simulink model "EHB_speedgoat_R2020a_V1"  (R2020a)
settings: Solver=FixedStepDiscrete  StartTime=0.0  StopTime=inf  FixedStep=0.001  RelTol=1e-3  EnableMultiTasking=on
model workspace (MAT data in the model file):
  A : Simulink.Signal (value not decoded)
  B : Simulink.Signal (value not decoded)
  C : Simulink.Signal (value not decoded)
  D : Simulink.Signal (value not decoded)
  E : Simulink.Signal (value not decoded)
  calin = [-9.96 -7.98 -5.98 -3.99 -1.994 0 1.995 3.992 5.99 7.98 9.97]
  calout = [-10 -8 -6 -4 -2 0 2 4 6 8 10]
symbols that are objects in the model workspace (value not decoded): C, D
undefined symbols (not defined in the file): Com1, none, ts_IO612
libraries: simulink x1436, xpcethercatlib x1223, yisutbxlib_utilities x256, xpcutilitieslib x156, hdlsllib x145, canmsglib x46, speedgoatlib_IO602_4 x11, speedgoatlib_IO611 x7, slrttcplib x4, CanManageLib x3, slrtlib x3, xpcseriallib x2
(part 19 of 30)

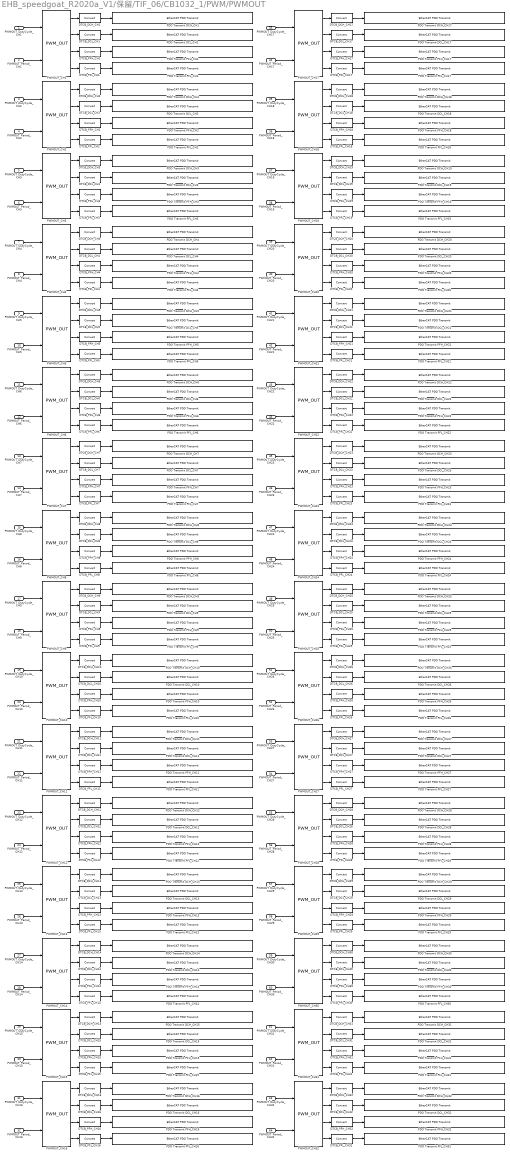
== system EHB_speedgoat_R2020a_V1/保留/TIF_06/CB1032_1/PWM/PWMOUT ==
  PWMOUT_DutyCycle_CH1 : Inport
  PWMOUT_Period_CH1 : Inport  Port=2
  PWMOUT_DutyCycle_CH2 : Inport  Port=3
  PWMOUT_Period_CH2 : Inport  Port=4
  PWMOUT_DutyCycle_CH3 : Inport  Port=5
  PWMOUT_Period_CH3 : Inport  Port=6
  PWMOUT_DutyCycle_CH4 : Inport  Port=7
  PWMOUT_Period_CH4 : Inport  Port=8
  PWMOUT_DutyCycle_CH5 : Inport  Port=9
  PWMOUT_Period_CH5 : Inport  Port=10
  PWMOUT_DutyCycle_CH6 : Inport  Port=11
  PWMOUT_Period_CH6 : Inport  Port=12
  PWMOUT_DutyCycle_CH7 : Inport  Port=13
  PWMOUT_Period_CH7 : Inport  Port=14
  PWMOUT_DutyCycle_CH8 : Inport  Port=15
  PWMOUT_Period_CH8 : Inport  Port=16
  PWMOUT_DutyCycle_CH9 : Inport  Port=17
  PWMOUT_Period_CH9 : Inport  Port=18
  PWMOUT_DutyCycle_CH10 : Inport  Port=19
  PWMOUT_Period_CH10 : Inport  Port=20
  PWMOUT_DutyCycle_CH11 : Inport  Port=21
  PWMOUT_Period_CH11 : Inport  Port=22
  PWMOUT_DutyCycle_CH12 : Inport  Port=23
  PWMOUT_Period_CH12 : Inport  Port=24
  PWMOUT_DutyCycle_CH13 : Inport  Port=25
  PWMOUT_Period_CH13 : Inport  Port=26
  PWMOUT_DutyCycle_CH14 : Inport  Port=27
  PWMOUT_Period_CH14 : Inport  Port=28
  PWMOUT_DutyCycle_CH15 : Inport  Port=29
  PWMOUT_Period_CH15 : Inport  Port=30
  PWMOUT_DutyCycle_CH16 : Inport  Port=31
  PWMOUT_Period_CH16 : Inport  Port=32
  PWMOUT_DutyCycle_CH17 : Inport  Port=33
  PWMOUT_Period_CH17 : Inport  Port=34
  PWMOUT_DutyCycle_CH18 : Inport  Port=35
  PWMOUT_Period_CH18 : Inport  Port=36
  PWMOUT_DutyCycle_CH19 : Inport  Port=37
  PWMOUT_Period_CH19 : Inport  Port=38
  PWMOUT_DutyCycle_CH20 : Inport  Port=39
  PWMOUT_Period_CH20 : Inport  Port=40
  PWMOUT_DutyCycle_CH21 : Inport  Port=41
  PWMOUT_Period_CH21 : Inport  Port=42
  PWMOUT_DutyCycle_CH22 : Inport  Port=43
  PWMOUT_Period_CH22 : Inport  Port=44
  PWMOUT_DutyCycle_CH23 : Inport  Port=45
  PWMOUT_Period_CH23 : Inport  Port=46
  PWMOUT_DutyCycle_CH24 : Inport  Port=47
  PWMOUT_Period_CH24 : Inport  Port=48
  PWMOUT_DutyCycle_CH25 : Inport  Port=49
  PWMOUT_Period_CH25 : Inport  Port=50
  PWMOUT_DutyCycle_CH26 : Inport  Port=51
  PWMOUT_Period_CH26 : Inport  Port=52
  PWMOUT_DutyCycle_CH27 : Inport  Port=53
  PWMOUT_Period_CH27 : Inport  Port=54
  PWMOUT_DutyCycle_CH28 : Inport  Port=55
  PWMOUT_Period_CH28 : Inport  Port=56
  PWMOUT_DutyCycle_CH29 : Inport  Port=57
  PWMOUT_Period_CH29 : Inport  Port=58
  PWMOUT_DutyCycle_CH30 : Inport  Port=59
  PWMOUT_Period_CH30 : Inport  Port=60
  PWMOUT_DutyCycle_CH31 : Inport  Port=61
  PWMOUT_Period_CH31 : Inport  Port=62
  PWMOUT_DutyCycle_CH32 : Inport  Port=63
  PWMOUT_Period_CH32 : Inport  Port=64
  DTCB_DCH_CH{1..32} (32 alike) : DataTypeConversion
  DTCB_DCL_CH{1..32} (32 alike) : DataTypeConversion
  DTCB_PFH_CH{1..32} (32 alike) : DataTypeConversion
  DTCB_PFL_CH{1..32} (32 alike) : DataTypeConversion
  PDO Transmit DCH_CH1 : xpcethercatlib/EtherCAT PDO Transmit   Priority=3  sig_name=Box 1 (YISUWORLD_Dig).PDOSet1 process data mapping.DCH1  sig_offset=376  sig_type=uint16  type_size=16  sig_dim=1  device_id=0  sample_time=0.001000
      settings: SourceProductBaseCode=XP
  PDO Transmit DCH_CH10 : xpcethercatlib/EtherCAT PDO Transmit   Priority=3  sig_name=Box 1 (YISUWORLD_Dig).PDOSet1 process data mapping.DCH10  sig_offset=520  sig_type=uint16  type_size=16  sig_dim=1  device_id=0  sample_time=0.001000
      settings: SourceProductBaseCode=XP
  PDO Transmit DCH_CH11 : xpcethercatlib/EtherCAT PDO Transmit   Priority=3  sig_name=Box 1 (YISUWORLD_Dig).PDOSet1 process data mapping.DCH11  sig_offset=536  sig_type=uint16  type_size=16  sig_dim=1  device_id=0  sample_time=0.001000
      settings: SourceProductBaseCode=XP
  PDO Transmit DCH_CH12 : xpcethercatlib/EtherCAT PDO Transmit   Priority=3  sig_name=Box 1 (YISUWORLD_Dig).PDOSet1 process data mapping.DCH12  sig_offset=552  sig_type=uint16  type_size=16  sig_dim=1  device_id=0  sample_time=0.001000
      settings: SourceProductBaseCode=XP
  PDO Transmit DCH_CH13 : xpcethercatlib/EtherCAT PDO Transmit   Priority=3  sig_name=Box 1 (YISUWORLD_Dig).PDOSet1 process data mapping.DCH13  sig_offset=568  sig_type=uint16  type_size=16  sig_dim=1  device_id=0  sample_time=0.001000
      settings: SourceProductBaseCode=XP
  PDO Transmit DCH_CH14 : xpcethercatlib/EtherCAT PDO Transmit   Priority=3  sig_name=Box 1 (YISUWORLD_Dig).PDOSet1 process data mapping.DCH14  sig_offset=584  sig_type=uint16  type_size=16  sig_dim=1  device_id=0  sample_time=0.001000
      settings: SourceProductBaseCode=XP
  PDO Transmit DCH_CH15 : xpcethercatlib/EtherCAT PDO Transmit   Priority=3  sig_name=Box 1 (YISUWORLD_Dig).PDOSet1 process data mapping.DCH15  sig_offset=600  sig_type=uint16  type_size=16  sig_dim=1  device_id=0  sample_time=0.001000
      settings: SourceProductBaseCode=XP
  PDO Transmit DCH_CH16 : xpcethercatlib/EtherCAT PDO Transmit   Priority=3  sig_name=Box 1 (YISUWORLD_Dig).PDOSet1 process data mapping.DCH16  sig_offset=616  sig_type=uint16  type_size=16  sig_dim=1  device_id=0  sample_time=0.001000
      settings: SourceProductBaseCode=XP
  PDO Transmit DCH_CH17 : xpcethercatlib/EtherCAT PDO Transmit   Priority=3  sig_name=Box 1 (YISUWORLD_Dig).PDOSet1 process data mapping.DCH17  sig_offset=632  sig_type=uint16  type_size=16  sig_dim=1  device_id=0  sample_time=0.001000
      settings: SourceProductBaseCode=XP
  PDO Transmit DCH_CH18 : xpcethercatlib/EtherCAT PDO Transmit   Priority=3  sig_name=Box 1 (YISUWORLD_Dig).PDOSet1 process data mapping.DCH18  sig_offset=648  sig_type=uint16  type_size=16  sig_dim=1  device_id=0  sample_time=0.001000
      settings: SourceProductBaseCode=XP
  PDO Transmit DCH_CH19 : xpcethercatlib/EtherCAT PDO Transmit   Priority=3  sig_name=Box 1 (YISUWORLD_Dig).PDOSet1 process data mapping.DCH19  sig_offset=664  sig_type=uint16  type_size=16  sig_dim=1  device_id=0  sample_time=0.001000
      settings: SourceProductBaseCode=XP
  PDO Transmit DCH_CH2 : xpcethercatlib/EtherCAT PDO Transmit   Priority=3  sig_name=Box 1 (YISUWORLD_Dig).PDOSet1 process data mapping.DCH2  sig_offset=392  sig_type=uint16  type_size=16  sig_dim=1  device_id=0  sample_time=0.001000
      settings: SourceProductBaseCode=XP
  PDO Transmit DCH_CH20 : xpcethercatlib/EtherCAT PDO Transmit   Priority=3  sig_name=Box 1 (YISUWORLD_Dig).PDOSet1 process data mapping.DCH20  sig_offset=680  sig_type=uint16  type_size=16  sig_dim=1  device_id=0  sample_time=0.001000
      settings: SourceProductBaseCode=XP
  PDO Transmit DCH_CH21 : xpcethercatlib/EtherCAT PDO Transmit   Priority=3  sig_name=Box 1 (YISUWORLD_Dig).PDOSet1 process data mapping.DCH21  sig_offset=696  sig_type=uint16  type_size=16  sig_dim=1  device_id=0  sample_time=0.001000
      settings: SourceProductBaseCode=XP
  PDO Transmit DCH_CH22 : xpcethercatlib/EtherCAT PDO Transmit   Priority=3  sig_name=Box 1 (YISUWORLD_Dig).PDOSet1 process data mapping.DCH22  sig_offset=712  sig_type=uint16  type_size=16  sig_dim=1  device_id=0  sample_time=0.001000
      settings: SourceProductBaseCode=XP
  PDO Transmit DCH_CH23 : xpcethercatlib/EtherCAT PDO Transmit   Priority=3  sig_name=Box 1 (YISUWORLD_Dig).PDOSet1 process data mapping.DCH23  sig_offset=728  sig_type=uint16  type_size=16  sig_dim=1  device_id=0  sample_time=0.001000
      settings: SourceProductBaseCode=XP
  PDO Transmit DCH_CH24 : xpcethercatlib/EtherCAT PDO Transmit   Priority=3  sig_name=Box 1 (YISUWORLD_Dig).PDOSet1 process data mapping.DCH24  sig_offset=744  sig_type=uint16  type_size=16  sig_dim=1  device_id=0  sample_time=0.001000
      settings: SourceProductBaseCode=XP
  PDO Transmit DCH_CH25 : xpcethercatlib/EtherCAT PDO Transmit   Priority=3  sig_name=Box 1 (YISUWORLD_Dig).PDOSet1 process data mapping.DCH25  sig_offset=760  sig_type=uint16  type_size=16  sig_dim=1  device_id=0  sample_time=0.001000
      settings: SourceProductBaseCode=XP
  PDO Transmit DCH_CH26 : xpcethercatlib/EtherCAT PDO Transmit   Priority=3  sig_name=Box 1 (YISUWORLD_Dig).PDOSet1 process data mapping.DCH26  sig_offset=776  sig_type=uint16  type_size=16  sig_dim=1  device_id=0  sample_time=0.001000
      settings: SourceProductBaseCode=XP
  PDO Transmit DCH_CH27 : xpcethercatlib/EtherCAT PDO Transmit   Priority=3  sig_name=Box 1 (YISUWORLD_Dig).PDOSet1 process data mapping.DCH27  sig_offset=792  sig_type=uint16  type_size=16  sig_dim=1  device_id=0  sample_time=0.001000
      settings: SourceProductBaseCode=XP
  PDO Transmit DCH_CH28 : xpcethercatlib/EtherCAT PDO Transmit   Priority=3  sig_name=Box 1 (YISUWORLD_Dig).PDOSet1 process data mapping.DCH28  sig_offset=808  sig_type=uint16  type_size=16  sig_dim=1  device_id=0  sample_time=0.001000
      settings: SourceProductBaseCode=XP
  PDO Transmit DCH_CH29 : xpcethercatlib/EtherCAT PDO Transmit   Priority=3  sig_name=Box 1 (YISUWORLD_Dig).PDOSet1 process data mapping.DCH29  sig_offset=824  sig_type=uint16  type_size=16  sig_dim=1  device_id=0  sample_time=0.001000
      settings: SourceProductBaseCode=XP
  PDO Transmit DCH_CH3 : xpcethercatlib/EtherCAT PDO Transmit   Priority=3  sig_name=Box 1 (YISUWORLD_Dig).PDOSet1 process data mapping.DCH3  sig_offset=408  sig_type=uint16  type_size=16  sig_dim=1  device_id=0  sample_time=0.001000
      settings: SourceProductBaseCode=XP
  PDO Transmit DCH_CH30 : xpcethercatlib/EtherCAT PDO Transmit   Priority=3  sig_name=Box 1 (YISUWORLD_Dig).PDOSet1 process data mapping.DCH30  sig_offset=840  sig_type=uint16  type_size=16  sig_dim=1  device_id=0  sample_time=0.001000
      settings: SourceProductBaseCode=XP
  PDO Transmit DCH_CH31 : xpcethercatlib/EtherCAT PDO Transmit   Priority=3  sig_name=Box 1 (YISUWORLD_Dig).PDOSet1 process data mapping.DCH31  sig_offset=856  sig_type=uint16  type_size=16  sig_dim=1  device_id=0  sample_time=0.001000
      settings: SourceProductBaseCode=XP
  PDO Transmit DCH_CH32 : xpcethercatlib/EtherCAT PDO Transmit   Priority=3  sig_name=Box 1 (YISUWORLD_Dig).PDOSet1 process data mapping.DCH32  sig_offset=872  sig_type=uint16  type_size=16  sig_dim=1  device_id=0  sample_time=0.001000
      settings: SourceProductBaseCode=XP
  PDO Transmit DCH_CH4 : xpcethercatlib/EtherCAT PDO Transmit   Priority=3  sig_name=Box 1 (YISUWORLD_Dig).PDOSet1 process data mapping.DCH4  sig_offset=424  sig_type=uint16  type_size=16  sig_dim=1  device_id=0  sample_time=0.001000
      settings: SourceProductBaseCode=XP
  PDO Transmit DCH_CH5 : xpcethercatlib/EtherCAT PDO Transmit   Priority=3  sig_name=Box 1 (YISUWORLD_Dig).PDOSet1 process data mapping.DCH5  sig_offset=440  sig_type=uint16  type_size=16  sig_dim=1  device_id=0  sample_time=0.001000
      settings: SourceProductBaseCode=XP
  PDO Transmit DCH_CH6 : xpcethercatlib/EtherCAT PDO Transmit   Priority=3  sig_name=Box 1 (YISUWORLD_Dig).PDOSet1 process data mapping.DCH6  sig_offset=456  sig_type=uint16  type_size=16  sig_dim=1  device_id=0  sample_time=0.001000
      settings: SourceProductBaseCode=XP
  PDO Transmit DCH_CH7 : xpcethercatlib/EtherCAT PDO Transmit   Priority=3  sig_name=Box 1 (YISUWORLD_Dig).PDOSet1 process data mapping.DCH7  sig_offset=472  sig_type=uint16  type_size=16  sig_dim=1  device_id=0  sample_time=0.001000
      settings: SourceProductBaseCode=XP
  PDO Transmit DCH_CH8 : xpcethercatlib/EtherCAT PDO Transmit   Priority=3  sig_name=Box 1 (YISUWORLD_Dig).PDOSet1 process data mapping.DCH8  sig_offset=488  sig_type=uint16  type_size=16  sig_dim=1  device_id=0  sample_time=0.001000
      settings: SourceProductBaseCode=XP
  PDO Transmit DCH_CH9 : xpcethercatlib/EtherCAT PDO Transmit   Priority=3  sig_name=Box 1 (YISUWORLD_Dig).PDOSet1 process data mapping.DCH9  sig_offset=504  sig_type=uint16  type_size=16  sig_dim=1  device_id=0  sample_time=0.001000
      settings: SourceProductBaseCode=XP
  PDO Transmit DCL_CH1 : xpcethercatlib/EtherCAT PDO Transmit   Priority=3  sig_name=Box 1 (YISUWORLD_Dig).PDOSet1 process data mapping.DCL1  sig_offset=888  sig_type=uint16  type_size=16  sig_dim=1  device_id=0  sample_time=0.001000
      settings: SourceProductBaseCode=XP
  PDO Transmit DCL_CH10 : xpcethercatlib/EtherCAT PDO Transmit   Priority=3  sig_name=Box 1 (YISUWORLD_Dig).PDOSet1 process data mapping.DCL10  sig_offset=1032  sig_type=uint16  type_size=16  sig_dim=1  device_id=0  sample_time=0.001000
      settings: SourceProductBaseCode=XP
  PDO Transmit DCL_CH11 : xpcethercatlib/EtherCAT PDO Transmit   Priority=3  sig_name=Box 1 (YISUWORLD_Dig).PDOSet1 process data mapping.DCL11  sig_offset=1048  sig_type=uint16  type_size=16  sig_dim=1  device_id=0  sample_time=0.001000
      settings: SourceProductBaseCode=XP
  PDO Transmit DCL_CH12 : xpcethercatlib/EtherCAT PDO Transmit   Priority=3  sig_name=Box 1 (YISUWORLD_Dig).PDOSet1 process data mapping.DCL12  sig_offset=1064  sig_type=uint16  type_size=16  sig_dim=1  device_id=0  sample_time=0.001000
      settings: SourceProductBaseCode=XP
  PDO Transmit DCL_CH13 : xpcethercatlib/EtherCAT PDO Transmit   Priority=3  sig_name=Box 1 (YISUWORLD_Dig).PDOSet1 process data mapping.DCL13  sig_offset=1080  sig_type=uint16  type_size=16  sig_dim=1  device_id=0  sample_time=0.001000
      settings: SourceProductBaseCode=XP
  PDO Transmit DCL_CH14 : xpcethercatlib/EtherCAT PDO Transmit   Priority=3  sig_name=Box 1 (YISUWORLD_Dig).PDOSet1 process data mapping.DCL14  sig_offset=1096  sig_type=uint16  type_size=16  sig_dim=1  device_id=0  sample_time=0.001000
      settings: SourceProductBaseCode=XP
  PDO Transmit DCL_CH15 : xpcethercatlib/EtherCAT PDO Transmit   Priority=3  sig_name=Box 1 (YISUWORLD_Dig).PDOSet1 process data mapping.DCL15  sig_offset=1112  sig_type=uint16  type_size=16  sig_dim=1  device_id=0  sample_time=0.001000
      settings: SourceProductBaseCode=XP
  PDO Transmit DCL_CH16 : xpcethercatlib/EtherCAT PDO Transmit   Priority=3  sig_name=Box 1 (YISUWORLD_Dig).PDOSet1 process data mapping.DCL16  sig_offset=1128  sig_type=uint16  type_size=16  sig_dim=1  device_id=0  sample_time=0.001000
      settings: SourceProductBaseCode=XP
  PDO Transmit DCL_CH17 : xpcethercatlib/EtherCAT PDO Transmit   Priority=3  sig_name=Box 1 (YISUWORLD_Dig).PDOSet1 process data mapping.DCL17  sig_offset=1144  sig_type=uint16  type_size=16  sig_dim=1  device_id=0  sample_time=0.001000
      settings: SourceProductBaseCode=XP
  PDO Transmit DCL_CH18 : xpcethercatlib/EtherCAT PDO Transmit   Priority=3  sig_name=Box 1 (YISUWORLD_Dig).PDOSet1 process data mapping.DCL18  sig_offset=1160  sig_type=uint16  type_size=16  sig_dim=1  device_id=0  sample_time=0.001000
      settings: SourceProductBaseCode=XP
  PDO Transmit DCL_CH19 : xpcethercatlib/EtherCAT PDO Transmit   Priority=3  sig_name=Box 1 (YISUWORLD_Dig).PDOSet1 process data mapping.DCL19  sig_offset=1176  sig_type=uint16  type_size=16  sig_dim=1  device_id=0  sample_time=0.001000
      settings: SourceProductBaseCode=XP
  PDO Transmit DCL_CH2 : xpcethercatlib/EtherCAT PDO Transmit   Priority=3  sig_name=Box 1 (YISUWORLD_Dig).PDOSet1 process data mapping.DCL2  sig_offset=904  sig_type=uint16  type_size=16  sig_dim=1  device_id=0  sample_time=0.001000
      settings: SourceProductBaseCode=XP
  PDO Transmit DCL_CH20 : xpcethercatlib/EtherCAT PDO Transmit   Priority=3  sig_name=Box 1 (YISUWORLD_Dig).PDOSet1 process data mapping.DCL20  sig_offset=1192  sig_type=uint16  type_size=16  sig_dim=1  device_id=0  sample_time=0.001000
      settings: SourceProductBaseCode=XP
  PDO Transmit DCL_CH21 : xpcethercatlib/EtherCAT PDO Transmit   Priority=3  sig_name=Box 1 (YISUWORLD_Dig).PDOSet1 process data mapping.DCL21  sig_offset=1208  sig_type=uint16  type_size=16  sig_dim=1  device_id=0  sample_time=0.001000
      settings: SourceProductBaseCode=XP
  PDO Transmit DCL_CH22 : xpcethercatlib/EtherCAT PDO Transmit   Priority=3  sig_name=Box 1 (YISUWORLD_Dig).PDOSet1 process data mapping.DCL22  sig_offset=1224  sig_type=uint16  type_size=16  sig_dim=1  device_id=0  sample_time=0.001000
      settings: SourceProductBaseCode=XP
  PDO Transmit DCL_CH23 : xpcethercatlib/EtherCAT PDO Transmit   Priority=3  sig_name=Box 1 (YISUWORLD_Dig).PDOSet1 process data mapping.DCL23  sig_offset=1240  sig_type=uint16  type_size=16  sig_dim=1  device_id=0  sample_time=0.001000
      settings: SourceProductBaseCode=XP
  PDO Transmit DCL_CH24 : xpcethercatlib/EtherCAT PDO Transmit   Priority=3  sig_name=Box 1 (YISUWORLD_Dig).PDOSet1 process data mapping.DCL24  sig_offset=1256  sig_type=uint16  type_size=16  sig_dim=1  device_id=0  sample_time=0.001000
      settings: SourceProductBaseCode=XP
  PDO Transmit DCL_CH25 : xpcethercatlib/EtherCAT PDO Transmit   Priority=3  sig_name=Box 1 (YISUWORLD_Dig).PDOSet1 process data mapping.DCL25  sig_offset=1272  sig_type=uint16  type_size=16  sig_dim=1  device_id=0  sample_time=0.001000
      settings: SourceProductBaseCode=XP
  PDO Transmit DCL_CH26 : xpcethercatlib/EtherCAT PDO Transmit   Priority=3  sig_name=Box 1 (YISUWORLD_Dig).PDOSet1 process data mapping.DCL26  sig_offset=1288  sig_type=uint16  type_size=16  sig_dim=1  device_id=0  sample_time=0.001000
      settings: SourceProductBaseCode=XP
  PDO Transmit DCL_CH27 : xpcethercatlib/EtherCAT PDO Transmit   Priority=3  sig_name=Box 1 (YISUWORLD_Dig).PDOSet1 process data mapping.DCL27  sig_offset=1304  sig_type=uint16  type_size=16  sig_dim=1  device_id=0  sample_time=0.001000
      settings: SourceProductBaseCode=XP
  PDO Transmit DCL_CH28 : xpcethercatlib/EtherCAT PDO Transmit   Priority=3  sig_name=Box 1 (YISUWORLD_Dig).PDOSet1 process data mapping.DCL28  sig_offset=1320  sig_type=uint16  type_size=16  sig_dim=1  device_id=0  sample_time=0.001000
      settings: SourceProductBaseCode=XP
  PDO Transmit DCL_CH29 : xpcethercatlib/EtherCAT PDO Transmit   Priority=3  sig_name=Box 1 (YISUWORLD_Dig).PDOSet1 process data mapping.DCL29  sig_offset=1336  sig_type=uint16  type_size=16  sig_dim=1  device_id=0  sample_time=0.001000
      settings: SourceProductBaseCode=XP
  PDO Transmit DCL_CH3 : xpcethercatlib/EtherCAT PDO Transmit   Priority=3  sig_name=Box 1 (YISUWORLD_Dig).PDOSet1 process data mapping.DCL3  sig_offset=920  sig_type=uint16  type_size=16  sig_dim=1  device_id=0  sample_time=0.001000
      settings: SourceProductBaseCode=XP
  PDO Transmit DCL_CH30 : xpcethercatlib/EtherCAT PDO Transmit   Priority=3  sig_name=Box 1 (YISUWORLD_Dig).PDOSet1 process data mapping.DCL30  sig_offset=1352  sig_type=uint16  type_size=16  sig_dim=1  device_id=0  sample_time=0.001000
      settings: SourceProductBaseCode=XP
  PDO Transmit DCL_CH31 : xpcethercatlib/EtherCAT PDO Transmit   Priority=3  sig_name=Box 1 (YISUWORLD_Dig).PDOSet1 process data mapping.DCL31  sig_offset=1368  sig_type=uint16  type_size=16  sig_dim=1  device_id=0  sample_time=0.001000
      settings: SourceProductBaseCode=XP
  PDO Transmit DCL_CH32 : xpcethercatlib/EtherCAT PDO Transmit   Priority=3  sig_name=Box 1 (YISUWORLD_Dig).PDOSet1 process data mapping.DCL32  sig_offset=1384  sig_type=uint16  type_size=16  sig_dim=1  device_id=0  sample_time=0.001000
      settings: SourceProductBaseCode=XP
  PDO Transmit DCL_CH4 : xpcethercatlib/EtherCAT PDO Transmit   Priority=3  sig_name=Box 1 (YISUWORLD_Dig).PDOSet1 process data mapping.DCL4  sig_offset=936  sig_type=uint16  type_size=16  sig_dim=1  device_id=0  sample_time=0.001000
      settings: SourceProductBaseCode=XP
  PDO Transmit DCL_CH5 : xpcethercatlib/EtherCAT PDO Transmit   Priority=3  sig_name=Box 1 (YISUWORLD_Dig).PDOSet1 process data mapping.DCL5  sig_offset=952  sig_type=uint16  type_size=16  sig_dim=1  device_id=0  sample_time=0.001000
      settings: SourceProductBaseCode=XP
  PDO Transmit DCL_CH6 : xpcethercatlib/EtherCAT PDO Transmit   Priority=3  sig_name=Box 1 (YISUWORLD_Dig).PDOSet1 process data mapping.DCL6  sig_offset=968  sig_type=uint16  type_size=16  sig_dim=1  device_id=0  sample_time=0.001000
      settings: SourceProductBaseCode=XP
  PDO Transmit DCL_CH7 : xpcethercatlib/EtherCAT PDO Transmit   Priority=3  sig_name=Box 1 (YISUWORLD_Dig).PDOSet1 process data mapping.DCL7  sig_offset=984  sig_type=uint16  type_size=16  sig_dim=1  device_id=0  sample_time=0.001000
      settings: SourceProductBaseCode=XP
  PDO Transmit DCL_CH8 : xpcethercatlib/EtherCAT PDO Transmit   Priority=3  sig_name=Box 1 (YISUWORLD_Dig).PDOSet1 process data mapping.DCL8  sig_offset=1000  sig_type=uint16  type_size=16  sig_dim=1  device_id=0  sample_time=0.001000
      settings: SourceProductBaseCode=XP
  PDO Transmit DCL_CH9 : xpcethercatlib/EtherCAT PDO Transmit   Priority=3  sig_name=Box 1 (YISUWORLD_Dig).PDOSet1 process data mapping.DCL9  sig_offset=1016  sig_type=uint16  type_size=16  sig_dim=1  device_id=0  sample_time=0.001000
      settings: SourceProductBaseCode=XP
  PDO Transmit PFH_CH1 : xpcethercatlib/EtherCAT PDO Transmit   Priority=3  sig_name=Box 1 (YISUWORLD_Dig).PDOSet1 process data mapping.PFH1  sig_offset=1400  sig_type=uint16  type_size=16  sig_dim=1  device_id=0  sample_time=0.001000
      settings: SourceProductBaseCode=XP
  PDO Transmit PFH_CH10 : xpcethercatlib/EtherCAT PDO Transmit   Priority=3  sig_name=Box 1 (YISUWORLD_Dig).PDOSet1 process data mapping.PFH10  sig_offset=1544  sig_type=uint16  type_size=16  sig_dim=1  device_id=0  sample_time=0.001000
      settings: SourceProductBaseCode=XP
  PDO Transmit PFH_CH11 : xpcethercatlib/EtherCAT PDO Transmit   Priority=3  sig_name=Box 1 (YISUWORLD_Dig).PDOSet1 process data mapping.PFH11  sig_offset=1560  sig_type=uint16  type_size=16  sig_dim=1  device_id=0  sample_time=0.001000
      settings: SourceProductBaseCode=XP
  PDO Transmit PFH_CH12 : xpcethercatlib/EtherCAT PDO Transmit   Priority=3  sig_name=Box 1 (YISUWORLD_Dig).PDOSet1 process data mapping.PFH12  sig_offset=1576  sig_type=uint16  type_size=16  sig_dim=1  device_id=0  sample_time=0.001000
      settings: SourceProductBaseCode=XP
  PDO Transmit PFH_CH13 : xpcethercatlib/EtherCAT PDO Transmit   Priority=3  sig_name=Box 1 (YISUWORLD_Dig).PDOSet1 process data mapping.PFH13  sig_offset=1592  sig_type=uint16  type_size=16  sig_dim=1  device_id=0  sample_time=0.001000
      settings: SourceProductBaseCode=XP
  PDO Transmit PFH_CH14 : xpcethercatlib/EtherCAT PDO Transmit   Priority=3  sig_name=Box 1 (YISUWORLD_Dig).PDOSet1 process data mapping.PFH14  sig_offset=1608  sig_type=uint16  type_size=16  sig_dim=1  device_id=0  sample_time=0.001000
      settings: SourceProductBaseCode=XP
  PDO Transmit PFH_CH15 : xpcethercatlib/EtherCAT PDO Transmit   Priority=3  sig_name=Box 1 (YISUWORLD_Dig).PDOSet1 process data mapping.PFH15  sig_offset=1624  sig_type=uint16  type_size=16  sig_dim=1  device_id=0  sample_time=0.001000
      settings: SourceProductBaseCode=XP
  PDO Transmit PFH_CH16 : xpcethercatlib/EtherCAT PDO Transmit   Priority=3  sig_name=Box 1 (YISUWORLD_Dig).PDOSet1 process data mapping.PFH16  sig_offset=1640  sig_type=uint16  type_size=16  sig_dim=1  device_id=0  sample_time=0.001000
      settings: SourceProductBaseCode=XP
  PDO Transmit PFH_CH17 : xpcethercatlib/EtherCAT PDO Transmit   Priority=3  sig_name=Box 1 (YISUWORLD_Dig).PDOSet1 process data mapping.PFH17  sig_offset=1656  sig_type=uint16  type_size=16  sig_dim=1  device_id=0  sample_time=0.001000
      settings: SourceProductBaseCode=XP
  PDO Transmit PFH_CH18 : xpcethercatlib/EtherCAT PDO Transmit   Priority=3  sig_name=Box 1 (YISUWORLD_Dig).PDOSet1 process data mapping.PFH18  sig_offset=1672  sig_type=uint16  type_size=16  sig_dim=1  device_id=0  sample_time=0.001000
      settings: SourceProductBaseCode=XP
  PDO Transmit PFH_CH19 : xpcethercatlib/EtherCAT PDO Transmit   Priority=3  sig_name=Box 1 (YISUWORLD_Dig).PDOSet1 process data mapping.PFH19  sig_offset=1688  sig_type=uint16  type_size=16  sig_dim=1  device_id=0  sample_time=0.001000
      settings: SourceProductBaseCode=XP
  PDO Transmit PFH_CH2 : xpcethercatlib/EtherCAT PDO Transmit   Priority=3  sig_name=Box 1 (YISUWORLD_Dig).PDOSet1 process data mapping.PFH2  sig_offset=1416  sig_type=uint16  type_size=16  sig_dim=1  device_id=0  sample_time=0.001000
      settings: SourceProductBaseCode=XP
  PDO Transmit PFH_CH20 : xpcethercatlib/EtherCAT PDO Transmit   Priority=3  sig_name=Box 1 (YISUWORLD_Dig).PDOSet1 process data mapping.PFH20  sig_offset=1704  sig_type=uint16  type_size=16  sig_dim=1  device_id=0  sample_time=0.001000
      settings: SourceProductBaseCode=XP
  PDO Transmit PFH_CH21 : xpcethercatlib/EtherCAT PDO Transmit   Priority=3  sig_name=Box 1 (YISUWORLD_Dig).PDOSet1 process data mapping.PFH21  sig_offset=1720  sig_type=uint16  type_size=16  sig_dim=1  device_id=0  sample_time=0.001000
      settings: SourceProductBaseCode=XP
  PDO Transmit PFH_CH22 : xpcethercatlib/EtherCAT PDO Transmit   Priority=3  sig_name=Box 1 (YISUWORLD_Dig).PDOSet1 process data mapping.PFH22  sig_offset=1736  sig_type=uint16  type_size=16  sig_dim=1  device_id=0  sample_time=0.001000
      settings: SourceProductBaseCode=XP
  PDO Transmit PFH_CH23 : xpcethercatlib/EtherCAT PDO Transmit   Priority=3  sig_name=Box 1 (YISUWORLD_Dig).PDOSet1 process data mapping.PFH23  sig_offset=1752  sig_type=uint16  type_size=16  sig_dim=1  device_id=0  sample_time=0.001000
      settings: SourceProductBaseCode=XP
  PDO Transmit PFH_CH24 : xpcethercatlib/EtherCAT PDO Transmit   Priority=3  sig_name=Box 1 (YISUWORLD_Dig).PDOSet1 process data mapping.PFH24  sig_offset=1768  sig_type=uint16  type_size=16  sig_dim=1  device_id=0  sample_time=0.001000
      settings: SourceProductBaseCode=XP
  PDO Transmit PFH_CH25 : xpcethercatlib/EtherCAT PDO Transmit   Priority=3  sig_name=Box 1 (YISUWORLD_Dig).PDOSet1 process data mapping.PFH25  sig_offset=1784  sig_type=uint16  type_size=16  sig_dim=1  device_id=0  sample_time=0.001000
      settings: SourceProductBaseCode=XP
  PDO Transmit PFH_CH26 : xpcethercatlib/EtherCAT PDO Transmit   Priority=3  sig_name=Box 1 (YISUWORLD_Dig).PDOSet1 process data mapping.PFH26  sig_offset=1800  sig_type=uint16  type_size=16  sig_dim=1  device_id=0  sample_time=0.001000
      settings: SourceProductBaseCode=XP
  PDO Transmit PFH_CH27 : xpcethercatlib/EtherCAT PDO Transmit   Priority=3  sig_name=Box 1 (YISUWORLD_Dig).PDOSet1 process data mapping.PFH27  sig_offset=1816  sig_type=uint16  type_size=16  sig_dim=1  device_id=0  sample_time=0.001000
      settings: SourceProductBaseCode=XP
  PDO Transmit PFH_CH28 : xpcethercatlib/EtherCAT PDO Transmit   Priority=3  sig_name=Box 1 (YISUWORLD_Dig).PDOSet1 process data mapping.PFH28  sig_offset=1832  sig_type=uint16  type_size=16  sig_dim=1  device_id=0  sample_time=0.001000
      settings: SourceProductBaseCode=XP
  PDO Transmit PFH_CH29 : xpcethercatlib/EtherCAT PDO Transmit   Priority=3  sig_name=Box 1 (YISUWORLD_Dig).PDOSet1 process data mapping.PFH29  sig_offset=1848  sig_type=uint16  type_size=16  sig_dim=1  device_id=0  sample_time=0.001000
      settings: SourceProductBaseCode=XP
  PDO Transmit PFH_CH3 : xpcethercatlib/EtherCAT PDO Transmit   Priority=3  sig_name=Box 1 (YISUWORLD_Dig).PDOSet1 process data mapping.PFH3  sig_offset=1432  sig_type=uint16  type_size=16  sig_dim=1  device_id=0  sample_time=0.001000
      settings: SourceProductBaseCode=XP
  PDO Transmit PFH_CH30 : xpcethercatlib/EtherCAT PDO Transmit   Priority=3  sig_name=Box 1 (YISUWORLD_Dig).PDOSet1 process data mapping.PFH30  sig_offset=1864  sig_type=uint16  type_size=16  sig_dim=1  device_id=0  sample_time=0.001000
      settings: SourceProductBaseCode=XP
  PDO Transmit PFH_CH31 : xpcethercatlib/EtherCAT PDO Transmit   Priority=3  sig_name=Box 1 (YISUWORLD_Dig).PDOSet1 process data mapping.PFH31  sig_offset=1880  sig_type=uint16  type_size=16  sig_dim=1  device_id=0  sample_time=0.001000
      settings: SourceProductBaseCode=XP
  PDO Transmit PFH_CH32 : xpcethercatlib/EtherCAT PDO Transmit   Priority=3  sig_name=Box 1 (YISUWORLD_Dig).PDOSet1 process data mapping.PFH32  sig_offset=1896  sig_type=uint16  type_size=16  sig_dim=1  device_id=0  sample_time=0.001000
      settings: SourceProductBaseCode=XP
  PDO Transmit PFH_CH4 : xpcethercatlib/EtherCAT PDO Transmit   Priority=3  sig_name=Box 1 (YISUWORLD_Dig).PDOSet1 process data mapping.PFH4  sig_offset=1448  sig_type=uint16  type_size=16  sig_dim=1  device_id=0  sample_time=0.001000
      settings: SourceProductBaseCode=XP
  PDO Transmit PFH_CH5 : xpcethercatlib/EtherCAT PDO Transmit   Priority=3  sig_name=Box 1 (YISUWORLD_Dig).PDOSet1 process data mapping.PFH5  sig_offset=1464  sig_type=uint16  type_size=16  sig_dim=1  device_id=0  sample_time=0.001000
      settings: SourceProductBaseCode=XP
  PDO Transmit PFH_CH6 : xpcethercatlib/EtherCAT PDO Transmit   Priority=3  sig_name=Box 1 (YISUWORLD_Dig).PDOSet1 process data mapping.PFH6  sig_offset=1480  sig_type=uint16  type_size=16  sig_dim=1  device_id=0  sample_time=0.001000
      settings: SourceProductBaseCode=XP
  PDO Transmit PFH_CH7 : xpcethercatlib/EtherCAT PDO Transmit   Priority=3  sig_name=Box 1 (YISUWORLD_Dig).PDOSet1 process data mapping.PFH7  sig_offset=1496  sig_type=uint16  type_size=16  sig_dim=1  device_id=0  sample_time=0.001000
      settings: SourceProductBaseCode=XP
  PDO Transmit PFH_CH8 : xpcethercatlib/EtherCAT PDO Transmit   Priority=3  sig_name=Box 1 (YISUWORLD_Dig).PDOSet1 process data mapping.PFH8  sig_offset=1512  sig_type=uint16  type_size=16  sig_dim=1  device_id=0  sample_time=0.001000
      settings: SourceProductBaseCode=XP
  PDO Transmit PFH_CH9 : xpcethercatlib/EtherCAT PDO Transmit   Priority=3  sig_name=Box 1 (YISUWORLD_Dig).PDOSet1 process data mapping.PFH9  sig_offset=1528  sig_type=uint16  type_size=16  sig_dim=1  device_id=0  sample_time=0.001000
      settings: SourceProductBaseCode=XP
  PDO Transmit PFL_CH1 : xpcethercatlib/EtherCAT PDO Transmit   Priority=3  sig_name=Box 1 (YISUWORLD_Dig).PDOSet1 process data mapping.PFL1  sig_offset=1912  sig_type=uint16  type_size=16  sig_dim=1  device_id=0  sample_time=0.001000
      settings: SourceProductBaseCode=XP
  PDO Transmit PFL_CH10 : xpcethercatlib/EtherCAT PDO Transmit   Priority=3  sig_name=Box 1 (YISUWORLD_Dig).PDOSet1 process data mapping.PFL10  sig_offset=2056  sig_type=uint16  type_size=16  sig_dim=1  device_id=0  sample_time=0.001000
      settings: SourceProductBaseCode=XP
  PDO Transmit PFL_CH11 : xpcethercatlib/EtherCAT PDO Transmit   Priority=3  sig_name=Box 1 (YISUWORLD_Dig).PDOSet1 process data mapping.PFL11  sig_offset=2072  sig_type=uint16  type_size=16  sig_dim=1  device_id=0  sample_time=0.001000
      settings: SourceProductBaseCode=XP
  PDO Transmit PFL_CH12 : xpcethercatlib/EtherCAT PDO Transmit   Priority=3  sig_name=Box 1 (YISUWORLD_Dig).PDOSet1 process data mapping.PFL12  sig_offset=2088  sig_type=uint16  type_size=16  sig_dim=1  device_id=0  sample_time=0.001000
      settings: SourceProductBaseCode=XP
  PDO Transmit PFL_CH13 : xpcethercatlib/EtherCAT PDO Transmit   Priority=3  sig_name=Box 1 (YISUWORLD_Dig).PDOSet1 process data mapping.PFL13  sig_offset=2104  sig_type=uint16  type_size=16  sig_dim=1  device_id=0  sample_time=0.001000
      settings: SourceProductBaseCode=XP
  PDO Transmit PFL_CH14 : xpcethercatlib/EtherCAT PDO Transmit   Priority=3  sig_name=Box 1 (YISUWORLD_Dig).PDOSet1 process data mapping.PFL14  sig_offset=2120  sig_type=uint16  type_size=16  sig_dim=1  device_id=0  sample_time=0.001000
      settings: SourceProductBaseCode=XP
  PDO Transmit PFL_CH15 : xpcethercatlib/EtherCAT PDO Transmit   Priority=3  sig_name=Box 1 (YISUWORLD_Dig).PDOSet1 process data mapping.PFL15  sig_offset=2136  sig_type=uint16  type_size=16  sig_dim=1  device_id=0  sample_time=0.001000
      settings: SourceProductBaseCode=XP
  PDO Transmit PFL_CH16 : xpcethercatlib/EtherCAT PDO Transmit   Priority=3  sig_name=Box 1 (YISUWORLD_Dig).PDOSet1 process data mapping.PFL16  sig_offset=2152  sig_type=uint16  type_size=16  sig_dim=1  device_id=0  sample_time=0.001000
      settings: SourceProductBaseCode=XP
  PDO Transmit PFL_CH17 : xpcethercatlib/EtherCAT PDO Transmit   Priority=3  sig_name=Box 1 (YISUWORLD_Dig).PDOSet1 process data mapping.PFL17  sig_offset=2168  sig_type=uint16  type_size=16  sig_dim=1  device_id=0  sample_time=0.001000
      settings: SourceProductBaseCode=XP
  PDO Transmit PFL_CH18 : xpcethercatlib/EtherCAT PDO Transmit   Priority=3  sig_name=Box 1 (YISUWORLD_Dig).PDOSet1 process data mapping.PFL18  sig_offset=2184  sig_type=uint16  type_size=16  sig_dim=1  device_id=0  sample_time=0.001000
      settings: SourceProductBaseCode=XP
  PDO Transmit PFL_CH19 : xpcethercatlib/EtherCAT PDO Transmit   Priority=3  sig_name=Box 1 (YISUWORLD_Dig).PDOSet1 process data mapping.PFL19  sig_offset=2200  sig_type=uint16  type_size=16  sig_dim=1  device_id=0  sample_time=0.001000
      settings: SourceProductBaseCode=XP
  PDO Transmit PFL_CH2 : xpcethercatlib/EtherCAT PDO Transmit   Priority=3  sig_name=Box 1 (YISUWORLD_Dig).PDOSet1 process data mapping.PFL2  sig_offset=1928  sig_type=uint16  type_size=16  sig_dim=1  device_id=0  sample_time=0.001000
      settings: SourceProductBaseCode=XP
  PDO Transmit PFL_CH20 : xpcethercatlib/EtherCAT PDO Transmit   Priority=3  sig_name=Box 1 (YISUWORLD_Dig).PDOSet1 process data mapping.PFL20  sig_offset=2216  sig_type=uint16  type_size=16  sig_dim=1  device_id=0  sample_time=0.001000
      settings: SourceProductBaseCode=XP
  PDO Transmit PFL_CH21 : xpcethercatlib/EtherCAT PDO Transmit   Priority=3  sig_name=Box 1 (YISUWORLD_Dig).PDOSet1 process data mapping.PFL21  sig_offset=2232  sig_type=uint16  type_size=16  sig_dim=1  device_id=0  sample_time=0.001000
      settings: SourceProductBaseCode=XP
  PDO Transmit PFL_CH22 : xpcethercatlib/EtherCAT PDO Transmit   Priority=3  sig_name=Box 1 (YISUWORLD_Dig).PDOSet1 process data mapping.PFL22  sig_offset=2248  sig_type=uint16  type_size=16  sig_dim=1  device_id=0  sample_time=0.001000
      settings: SourceProductBaseCode=XP
  PDO Transmit PFL_CH23 : xpcethercatlib/EtherCAT PDO Transmit   Priority=3  sig_name=Box 1 (YISUWORLD_Dig).PDOSet1 process data mapping.PFL23  sig_offset=2264  sig_type=uint16  type_size=16  sig_dim=1  device_id=0  sample_time=0.001000
      settings: SourceProductBaseCode=XP
  PDO Transmit PFL_CH24 : xpcethercatlib/EtherCAT PDO Transmit   Priority=3  sig_name=Box 1 (YISUWORLD_Dig).PDOSet1 process data mapping.PFL24  sig_offset=2280  sig_type=uint16  type_size=16  sig_dim=1  device_id=0  sample_time=0.001000
      settings: SourceProductBaseCode=XP
  PDO Transmit PFL_CH25 : xpcethercatlib/EtherCAT PDO Transmit   Priority=3  sig_name=Box 1 (YISUWORLD_Dig).PDOSet1 process data mapping.PFL25  sig_offset=2296  sig_type=uint16  type_size=16  sig_dim=1  device_id=0  sample_time=0.001000
      settings: SourceProductBaseCode=XP
  PDO Transmit PFL_CH26 : xpcethercatlib/EtherCAT PDO Transmit   Priority=3  sig_name=Box 1 (YISUWORLD_Dig).PDOSet1 process data mapping.PFL26  sig_offset=2312  sig_type=uint16  type_size=16  sig_dim=1  device_id=0  sample_time=0.001000
      settings: SourceProductBaseCode=XP
  PDO Transmit PFL_CH27 : xpcethercatlib/EtherCAT PDO Transmit   Priority=3  sig_name=Box 1 (YISUWORLD_Dig).PDOSet1 process data mapping.PFL27  sig_offset=2328  sig_type=uint16  type_size=16  sig_dim=1  device_id=0  sample_time=0.001000
      settings: SourceProductBaseCode=XP
  PDO Transmit PFL_CH28 : xpcethercatlib/EtherCAT PDO Transmit   Priority=3  sig_name=Box 1 (YISUWORLD_Dig).PDOSet1 process data mapping.PFL28  sig_offset=2344  sig_type=uint16  type_size=16  sig_dim=1  device_id=0  sample_time=0.001000
      settings: SourceProductBaseCode=XP
  PDO Transmit PFL_CH29 : xpcethercatlib/EtherCAT PDO Transmit   Priority=3  sig_name=Box 1 (YISUWORLD_Dig).PDOSet1 process data mapping.PFL29  sig_offset=2360  sig_type=uint16  type_size=16  sig_dim=1  device_id=0  sample_time=0.001000
      settings: SourceProductBaseCode=XP
  PDO Transmit PFL_CH3 : xpcethercatlib/EtherCAT PDO Transmit   Priority=3  sig_name=Box 1 (YISUWORLD_Dig).PDOSet1 process data mapping.PFL3  sig_offset=1944  sig_type=uint16  type_size=16  sig_dim=1  device_id=0  sample_time=0.001000
      settings: SourceProductBaseCode=XP
  PDO Transmit PFL_CH30 : xpcethercatlib/EtherCAT PDO Transmit   Priority=3  sig_name=Box 1 (YISUWORLD_Dig).PDOSet1 process data mapping.PFL30  sig_offset=2376  sig_type=uint16  type_size=16  sig_dim=1  device_id=0  sample_time=0.001000
      settings: SourceProductBaseCode=XP
  PDO Transmit PFL_CH31 : xpcethercatlib/EtherCAT PDO Transmit   Priority=3  sig_name=Box 1 (YISUWORLD_Dig).PDOSet1 process data mapping.PFL31  sig_offset=2392  sig_type=uint16  type_size=16  sig_dim=1  device_id=0  sample_time=0.001000
      settings: SourceProductBaseCode=XP
  PDO Transmit PFL_CH32 : xpcethercatlib/EtherCAT PDO Transmit   Priority=3  sig_name=Box 1 (YISUWORLD_Dig).PDOSet1 process data mapping.PFL32  sig_offset=2408  sig_type=uint16  type_size=16  sig_dim=1  device_id=0  sample_time=0.001000
      settings: SourceProductBaseCode=XP
  PDO Transmit PFL_CH4 : xpcethercatlib/EtherCAT PDO Transmit   Priority=3  sig_name=Box 1 (YISUWORLD_Dig).PDOSet1 process data mapping.PFL4  sig_offset=1960  sig_type=uint16  type_size=16  sig_dim=1  device_id=0  sample_time=0.001000
      settings: SourceProductBaseCode=XP
  PDO Transmit PFL_CH5 : xpcethercatlib/EtherCAT PDO Transmit   Priority=3  sig_name=Box 1 (YISUWORLD_Dig).PDOSet1 process data mapping.PFL5  sig_offset=1976  sig_type=uint16  type_size=16  sig_dim=1  device_id=0  sample_time=0.001000
      settings: SourceProductBaseCode=XP
  PDO Transmit PFL_CH6 : xpcethercatlib/EtherCAT PDO Transmit   Priority=3  sig_name=Box 1 (YISUWORLD_Dig).PDOSet1 process data mapping.PFL6  sig_offset=1992  sig_type=uint16  type_size=16  sig_dim=1  device_id=0  sample_time=0.001000
      settings: SourceProductBaseCode=XP
  PDO Transmit PFL_CH7 : xpcethercatlib/EtherCAT PDO Transmit   Priority=3  sig_name=Box 1 (YISUWORLD_Dig).PDOSet1 process data mapping.PFL7  sig_offset=2008  sig_type=uint16  type_size=16  sig_dim=1  device_id=0  sample_time=0.001000
      settings: SourceProductBaseCode=XP
  PDO Transmit PFL_CH8 : xpcethercatlib/EtherCAT PDO Transmit   Priority=3  sig_name=Box 1 (YISUWORLD_Dig).PDOSet1 process data mapping.PFL8  sig_offset=2024  sig_type=uint16  type_size=16  sig_dim=1  device_id=0  sample_time=0.001000
      settings: SourceProductBaseCode=XP
  PDO Transmit PFL_CH9 : xpcethercatlib/EtherCAT PDO Transmit   Priority=3  sig_name=Box 1 (YISUWORLD_Dig).PDOSet1 process data mapping.PFL9  sig_offset=2040  sig_type=uint16  type_size=16  sig_dim=1  device_id=0  sample_time=0.001000
      settings: SourceProductBaseCode=XP
  PWMOUT_CH{1..32} (32 alike) : yisutbxlib_utilities/PWM_OUT  SystemSampleTime=-1  Latency=0  AutoFrameSizeCalculation=off
      settings: SourceProductName=YISU Toolbox Library
  wires:
  PWMOUT_DutyCycle_CH1/1 -> PWMOUT_CH1/1
  PWMOUT_Period_CH1/1 -> PWMOUT_CH1/2
  PWMOUT_CH1/1 -> DTCB_DCH_CH1/1
  DTCB_DCH_CH1/1 -> PDO Transmit DCH_CH1/1
  PWMOUT_CH1/2 -> DTCB_DCL_CH1/1
  DTCB_DCL_CH1/1 -> PDO Transmit DCL_CH1/1
  PWMOUT_CH1/3 -> DTCB_PFH_CH1/1
  DTCB_PFH_CH1/1 -> PDO Transmit PFH_CH1/1
  PWMOUT_CH1/4 -> DTCB_PFL_CH1/1
  DTCB_PFL_CH1/1 -> PDO Transmit PFL_CH1/1
  PWMOUT_DutyCycle_CH2/1 -> PWMOUT_CH2/1
  PWMOUT_Period_CH2/1 -> PWMOUT_CH2/2
  PWMOUT_CH2/1 -> DTCB_DCH_CH2/1
  DTCB_DCH_CH2/1 -> PDO Transmit DCH_CH2/1
  PWMOUT_CH2/2 -> DTCB_DCL_CH2/1
  DTCB_DCL_CH2/1 -> PDO Transmit DCL_CH2/1
  PWMOUT_CH2/3 -> DTCB_PFH_CH2/1
  DTCB_PFH_CH2/1 -> PDO Transmit PFH_CH2/1
  PWMOUT_CH2/4 -> DTCB_PFL_CH2/1
  DTCB_PFL_CH2/1 -> PDO Transmit PFL_CH2/1
  PWMOUT_DutyCycle_CH3/1 -> PWMOUT_CH3/1
  PWMOUT_Period_CH3/1 -> PWMOUT_CH3/2
  PWMOUT_CH3/1 -> DTCB_DCH_CH3/1
  DTCB_DCH_CH3/1 -> PDO Transmit DCH_CH3/1
  PWMOUT_CH3/2 -> DTCB_DCL_CH3/1
  DTCB_DCL_CH3/1 -> PDO Transmit DCL_CH3/1
  PWMOUT_CH3/3 -> DTCB_PFH_CH3/1
  DTCB_PFH_CH3/1 -> PDO Transmit PFH_CH3/1
  PWMOUT_CH3/4 -> DTCB_PFL_CH3/1
  DTCB_PFL_CH3/1 -> PDO Transmit PFL_CH3/1
  PWMOUT_DutyCycle_CH4/1 -> PWMOUT_CH4/1
  PWMOUT_Period_CH4/1 -> PWMOUT_CH4/2
  PWMOUT_CH4/1 -> DTCB_DCH_CH4/1
  DTCB_DCH_CH4/1 -> PDO Transmit DCH_CH4/1
  PWMOUT_CH4/2 -> DTCB_DCL_CH4/1
  DTCB_DCL_CH4/1 -> PDO Transmit DCL_CH4/1
  PWMOUT_CH4/3 -> DTCB_PFH_CH4/1
  DTCB_PFH_CH4/1 -> PDO Transmit PFH_CH4/1
  PWMOUT_CH4/4 -> DTCB_PFL_CH4/1
  DTCB_PFL_CH4/1 -> PDO Transmit PFL_CH4/1
  PWMOUT_DutyCycle_CH5/1 -> PWMOUT_CH5/1
  PWMOUT_Period_CH5/1 -> PWMOUT_CH5/2
  PWMOUT_CH5/1 -> DTCB_DCH_CH5/1
  DTCB_DCH_CH5/1 -> PDO Transmit DCH_CH5/1
  PWMOUT_CH5/2 -> DTCB_DCL_CH5/1
  DTCB_DCL_CH5/1 -> PDO Transmit DCL_CH5/1
  PWMOUT_CH5/3 -> DTCB_PFH_CH5/1
  DTCB_PFH_CH5/1 -> PDO Transmit PFH_CH5/1
  PWMOUT_CH5/4 -> DTCB_PFL_CH5/1
  DTCB_PFL_CH5/1 -> PDO Transmit PFL_CH5/1
  PWMOUT_DutyCycle_CH6/1 -> PWMOUT_CH6/1
  PWMOUT_Period_CH6/1 -> PWMOUT_CH6/2
  PWMOUT_CH6/1 -> DTCB_DCH_CH6/1
  DTCB_DCH_CH6/1 -> PDO Transmit DCH_CH6/1
  PWMOUT_CH6/2 -> DTCB_DCL_CH6/1
  DTCB_DCL_CH6/1 -> PDO Transmit DCL_CH6/1
  PWMOUT_CH6/3 -> DTCB_PFH_CH6/1
  DTCB_PFH_CH6/1 -> PDO Transmit PFH_CH6/1
  PWMOUT_CH6/4 -> DTCB_PFL_CH6/1
  DTCB_PFL_CH6/1 -> PDO Transmit PFL_CH6/1
  PWMOUT_DutyCycle_CH7/1 -> PWMOUT_CH7/1
  PWMOUT_Period_CH7/1 -> PWMOUT_CH7/2
  PWMOUT_CH7/1 -> DTCB_DCH_CH7/1
  DTCB_DCH_CH7/1 -> PDO Transmit DCH_CH7/1
  PWMOUT_CH7/2 -> DTCB_DCL_CH7/1
  DTCB_DCL_CH7/1 -> PDO Transmit DCL_CH7/1
  PWMOUT_CH7/3 -> DTCB_PFH_CH7/1
  DTCB_PFH_CH7/1 -> PDO Transmit PFH_CH7/1
  PWMOUT_CH7/4 -> DTCB_PFL_CH7/1
  DTCB_PFL_CH7/1 -> PDO Transmit PFL_CH7/1
  PWMOUT_DutyCycle_CH8/1 -> PWMOUT_CH8/1
  PWMOUT_Period_CH8/1 -> PWMOUT_CH8/2
  PWMOUT_CH8/1 -> DTCB_DCH_CH8/1
  DTCB_DCH_CH8/1 -> PDO Transmit DCH_CH8/1
  PWMOUT_CH8/2 -> DTCB_DCL_CH8/1
  DTCB_DCL_CH8/1 -> PDO Transmit DCL_CH8/1
  PWMOUT_CH8/3 -> DTCB_PFH_CH8/1
  DTCB_PFH_CH8/1 -> PDO Transmit PFH_CH8/1
  PWMOUT_CH8/4 -> DTCB_PFL_CH8/1
  DTCB_PFL_CH8/1 -> PDO Transmit PFL_CH8/1
  PWMOUT_DutyCycle_CH9/1 -> PWMOUT_CH9/1
  PWMOUT_Period_CH9/1 -> PWMOUT_CH9/2
  PWMOUT_CH9/1 -> DTCB_DCH_CH9/1
  DTCB_DCH_CH9/1 -> PDO Transmit DCH_CH9/1
  PWMOUT_CH9/2 -> DTCB_DCL_CH9/1
  DTCB_DCL_CH9/1 -> PDO Transmit DCL_CH9/1
  PWMOUT_CH9/3 -> DTCB_PFH_CH9/1
  DTCB_PFH_CH9/1 -> PDO Transmit PFH_CH9/1
  PWMOUT_CH9/4 -> DTCB_PFL_CH9/1
  DTCB_PFL_CH9/1 -> PDO Transmit PFL_CH9/1
  PWMOUT_DutyCycle_CH10/1 -> PWMOUT_CH10/1
  PWMOUT_Period_CH10/1 -> PWMOUT_CH10/2
  PWMOUT_CH10/1 -> DTCB_DCH_CH10/1
  DTCB_DCH_CH10/1 -> PDO Transmit DCH_CH10/1
  PWMOUT_CH10/2 -> DTCB_DCL_CH10/1
  DTCB_DCL_CH10/1 -> PDO Transmit DCL_CH10/1
  PWMOUT_CH10/3 -> DTCB_PFH_CH10/1
  DTCB_PFH_CH10/1 -> PDO Transmit PFH_CH10/1
  PWMOUT_CH10/4 -> DTCB_PFL_CH10/1
  DTCB_PFL_CH10/1 -> PDO Transmit PFL_CH10/1
  PWMOUT_DutyCycle_CH11/1 -> PWMOUT_CH11/1
  PWMOUT_Period_CH11/1 -> PWMOUT_CH11/2
  PWMOUT_CH11/1 -> DTCB_DCH_CH11/1
  DTCB_DCH_CH11/1 -> PDO Transmit DCH_CH11/1
  PWMOUT_CH11/2 -> DTCB_DCL_CH11/1
  DTCB_DCL_CH11/1 -> PDO Transmit DCL_CH11/1
  PWMOUT_CH11/3 -> DTCB_PFH_CH11/1
  DTCB_PFH_CH11/1 -> PDO Transmit PFH_CH11/1
  PWMOUT_CH11/4 -> DTCB_PFL_CH11/1
  DTCB_PFL_CH11/1 -> PDO Transmit PFL_CH11/1
  PWMOUT_DutyCycle_CH12/1 -> PWMOUT_CH12/1
  PWMOUT_Period_CH12/1 -> PWMOUT_CH12/2
  PWMOUT_CH12/1 -> DTCB_DCH_CH12/1
  DTCB_DCH_CH12/1 -> PDO Transmit DCH_CH12/1
  PWMOUT_CH12/2 -> DTCB_DCL_CH12/1
  DTCB_DCL_CH12/1 -> PDO Transmit DCL_CH12/1
  PWMOUT_CH12/3 -> DTCB_PFH_CH12/1
  DTCB_PFH_CH12/1 -> PDO Transmit PFH_CH12/1
  PWMOUT_CH12/4 -> DTCB_PFL_CH12/1
  DTCB_PFL_CH12/1 -> PDO Transmit PFL_CH12/1
  PWMOUT_DutyCycle_CH13/1 -> PWMOUT_CH13/1
  PWMOUT_Period_CH13/1 -> PWMOUT_CH13/2
  PWMOUT_CH13/1 -> DTCB_DCH_CH13/1
  DTCB_DCH_CH13/1 -> PDO Transmit DCH_CH13/1
  PWMOUT_CH13/2 -> DTCB_DCL_CH13/1
  DTCB_DCL_CH13/1 -> PDO Transmit DCL_CH13/1
  PWMOUT_CH13/3 -> DTCB_PFH_CH13/1
  DTCB_PFH_CH13/1 -> PDO Transmit PFH_CH13/1
  PWMOUT_CH13/4 -> DTCB_PFL_CH13/1
  DTCB_PFL_CH13/1 -> PDO Transmit PFL_CH13/1
  PWMOUT_DutyCycle_CH14/1 -> PWMOUT_CH14/1
  PWMOUT_Period_CH14/1 -> PWMOUT_CH14/2
  PWMOUT_CH14/1 -> DTCB_DCH_CH14/1
  DTCB_DCH_CH14/1 -> PDO Transmit DCH_CH14/1
  PWMOUT_CH14/2 -> DTCB_DCL_CH14/1
  DTCB_DCL_CH14/1 -> PDO Transmit DCL_CH14/1
  PWMOUT_CH14/3 -> DTCB_PFH_CH14/1
  DTCB_PFH_CH14/1 -> PDO Transmit PFH_CH14/1
  PWMOUT_CH14/4 -> DTCB_PFL_CH14/1
  DTCB_PFL_CH14/1 -> PDO Transmit PFL_CH14/1
  PWMOUT_DutyCycle_CH15/1 -> PWMOUT_CH15/1
  PWMOUT_Period_CH15/1 -> PWMOUT_CH15/2
  PWMOUT_CH15/1 -> DTCB_DCH_CH15/1
  DTCB_DCH_CH15/1 -> PDO Transmit DCH_CH15/1
  PWMOUT_CH15/2 -> DTCB_DCL_CH15/1
  DTCB_DCL_CH15/1 -> PDO Transmit DCL_CH15/1
  PWMOUT_CH15/3 -> DTCB_PFH_CH15/1
  DTCB_PFH_CH15/1 -> PDO Transmit PFH_CH15/1
  PWMOUT_CH15/4 -> DTCB_PFL_CH15/1
  DTCB_PFL_CH15/1 -> PDO Transmit PFL_CH15/1
  PWMOUT_DutyCycle_CH16/1 -> PWMOUT_CH16/1
  PWMOUT_Period_CH16/1 -> PWMOUT_CH16/2
  PWMOUT_CH16/1 -> DTCB_DCH_CH16/1
  DTCB_DCH_CH16/1 -> PDO Transmit DCH_CH16/1
  PWMOUT_CH16/2 -> DTCB_DCL_CH16/1
  DTCB_DCL_CH16/1 -> PDO Transmit DCL_CH16/1
  PWMOUT_CH16/3 -> DTCB_PFH_CH16/1
  DTCB_PFH_CH16/1 -> PDO Transmit PFH_CH16/1
  PWMOUT_CH16/4 -> DTCB_PFL_CH16/1
  DTCB_PFL_CH16/1 -> PDO Transmit PFL_CH16/1
  PWMOUT_DutyCycle_CH17/1 -> PWMOUT_CH17/1
  PWMOUT_Period_CH17/1 -> PWMOUT_CH17/2
  PWMOUT_CH17/1 -> DTCB_DCH_CH17/1
  DTCB_DCH_CH17/1 -> PDO Transmit DCH_CH17/1
  PWMOUT_CH17/2 -> DTCB_DCL_CH17/1
  DTCB_DCL_CH17/1 -> PDO Transmit DCL_CH17/1
  PWMOUT_CH17/3 -> DTCB_PFH_CH17/1
  DTCB_PFH_CH17/1 -> PDO Transmit PFH_CH17/1
  PWMOUT_CH17/4 -> DTCB_PFL_CH17/1
  DTCB_PFL_CH17/1 -> PDO Transmit PFL_CH17/1
  PWMOUT_DutyCycle_CH18/1 -> PWMOUT_CH18/1
  PWMOUT_Period_CH18/1 -> PWMOUT_CH18/2
  PWMOUT_CH18/1 -> DTCB_DCH_CH18/1
  DTCB_DCH_CH18/1 -> PDO Transmit DCH_CH18/1
  PWMOUT_CH18/2 -> DTCB_DCL_CH18/1
  DTCB_DCL_CH18/1 -> PDO Transmit DCL_CH18/1
  PWMOUT_CH18/3 -> DTCB_PFH_CH18/1
  DTCB_PFH_CH18/1 -> PDO Transmit PFH_CH18/1
  PWMOUT_CH18/4 -> DTCB_PFL_CH18/1
  DTCB_PFL_CH18/1 -> PDO Transmit PFL_CH18/1
  PWMOUT_DutyCycle_CH19/1 -> PWMOUT_CH19/1
  PWMOUT_Period_CH19/1 -> PWMOUT_CH19/2
  PWMOUT_CH19/1 -> DTCB_DCH_CH19/1
  DTCB_DCH_CH19/1 -> PDO Transmit DCH_CH19/1
  PWMOUT_CH19/2 -> DTCB_DCL_CH19/1
  DTCB_DCL_CH19/1 -> PDO Transmit DCL_CH19/1
  PWMOUT_CH19/3 -> DTCB_PFH_CH19/1
  DTCB_PFH_CH19/1 -> PDO Transmit PFH_CH19/1
  PWMOUT_CH19/4 -> DTCB_PFL_CH19/1
  DTCB_PFL_CH19/1 -> PDO Transmit PFL_CH19/1
  PWMOUT_DutyCycle_CH20/1 -> PWMOUT_CH20/1
  PWMOUT_Period_CH20/1 -> PWMOUT_CH20/2
  PWMOUT_CH20/1 -> DTCB_DCH_CH20/1
  DTCB_DCH_CH20/1 -> PDO Transmit DCH_CH20/1
  PWMOUT_CH20/2 -> DTCB_DCL_CH20/1
  DTCB_DCL_CH20/1 -> PDO Transmit DCL_CH20/1
  PWMOUT_CH20/3 -> DTCB_PFH_CH20/1
  DTCB_PFH_CH20/1 -> PDO Transmit PFH_CH20/1
  PWMOUT_CH20/4 -> DTCB_PFL_CH20/1
  DTCB_PFL_CH20/1 -> PDO Transmit PFL_CH20/1
  PWMOUT_DutyCycle_CH21/1 -> PWMOUT_CH21/1
  PWMOUT_Period_CH21/1 -> PWMOUT_CH21/2
  PWMOUT_CH21/1 -> DTCB_DCH_CH21/1
  DTCB_DCH_CH21/1 -> PDO Transmit DCH_CH21/1
  PWMOUT_CH21/2 -> DTCB_DCL_CH21/1
  DTCB_DCL_CH21/1 -> PDO Transmit DCL_CH21/1
  PWMOUT_CH21/3 -> DTCB_PFH_CH21/1
  DTCB_PFH_CH21/1 -> PDO Transmit PFH_CH21/1
  PWMOUT_CH21/4 -> DTCB_PFL_CH21/1
  DTCB_PFL_CH21/1 -> PDO Transmit PFL_CH21/1
  PWMOUT_DutyCycle_CH22/1 -> PWMOUT_CH22/1
  PWMOUT_Period_CH22/1 -> PWMOUT_CH22/2
  PWMOUT_CH22/1 -> DTCB_DCH_CH22/1
  DTCB_DCH_CH22/1 -> PDO Transmit DCH_CH22/1
  PWMOUT_CH22/2 -> DTCB_DCL_CH22/1
  DTCB_DCL_CH22/1 -> PDO Transmit DCL_CH22/1
  PWMOUT_CH22/3 -> DTCB_PFH_CH22/1
  DTCB_PFH_CH22/1 -> PDO Transmit PFH_CH22/1
  PWMOUT_CH22/4 -> DTCB_PFL_CH22/1
  DTCB_PFL_CH22/1 -> PDO Transmit PFL_CH22/1
  PWMOUT_DutyCycle_CH23/1 -> PWMOUT_CH23/1
  PWMOUT_Period_CH23/1 -> PWMOUT_CH23/2
  PWMOUT_CH23/1 -> DTCB_DCH_CH23/1
  DTCB_DCH_CH23/1 -> PDO Transmit DCH_CH23/1
  PWMOUT_CH23/2 -> DTCB_DCL_CH23/1
  DTCB_DCL_CH23/1 -> PDO Transmit DCL_CH23/1
  PWMOUT_CH23/3 -> DTCB_PFH_CH23/1
  DTCB_PFH_CH23/1 -> PDO Transmit PFH_CH23/1
  PWMOUT_CH23/4 -> DTCB_PFL_CH23/1
  DTCB_PFL_CH23/1 -> PDO Transmit PFL_CH23/1
  PWMOUT_DutyCycle_CH24/1 -> PWMOUT_CH24/1
  PWMOUT_Period_CH24/1 -> PWMOUT_CH24/2
  PWMOUT_CH24/1 -> DTCB_DCH_CH24/1
  DTCB_DCH_CH24/1 -> PDO Transmit DCH_CH24/1
  PWMOUT_CH24/2 -> DTCB_DCL_CH24/1
  DTCB_DCL_CH24/1 -> PDO Transmit DCL_CH24/1
  PWMOUT_CH24/3 -> DTCB_PFH_CH24/1
  DTCB_PFH_CH24/1 -> PDO Transmit PFH_CH24/1
  PWMOUT_CH24/4 -> DTCB_PFL_CH24/1
  DTCB_PFL_CH24/1 -> PDO Transmit PFL_CH24/1
  PWMOUT_DutyCycle_CH25/1 -> PWMOUT_CH25/1
  PWMOUT_Period_CH25/1 -> PWMOUT_CH25/2
  PWMOUT_CH25/1 -> DTCB_DCH_CH25/1
  DTCB_DCH_CH25/1 -> PDO Transmit DCH_CH25/1
  PWMOUT_CH25/2 -> DTCB_DCL_CH25/1
  DTCB_DCL_CH25/1 -> PDO Transmit DCL_CH25/1
  PWMOUT_CH25/3 -> DTCB_PFH_CH25/1
  DTCB_PFH_CH25/1 -> PDO Transmit PFH_CH25/1
  PWMOUT_CH25/4 -> DTCB_PFL_CH25/1
  DTCB_PFL_CH25/1 -> PDO Transmit PFL_CH25/1
  PWMOUT_DutyCycle_CH26/1 -> PWMOUT_CH26/1
  PWMOUT_Period_CH26/1 -> PWMOUT_CH26/2
  PWMOUT_CH26/1 -> DTCB_DCH_CH26/1
  DTCB_DCH_CH26/1 -> PDO Transmit DCH_CH26/1
  PWMOUT_CH26/2 -> DTCB_DCL_CH26/1
  DTCB_DCL_CH26/1 -> PDO Transmit DCL_CH26/1
  PWMOUT_CH26/3 -> DTCB_PFH_CH26/1
  DTCB_PFH_CH26/1 -> PDO Transmit PFH_CH26/1
  PWMOUT_CH26/4 -> DTCB_PFL_CH26/1
  DTCB_PFL_CH26/1 -> PDO Transmit PFL_CH26/1
  PWMOUT_DutyCycle_CH27/1 -> PWMOUT_CH27/1
  PWMOUT_Period_CH27/1 -> PWMOUT_CH27/2
  PWMOUT_CH27/1 -> DTCB_DCH_CH27/1
  DTCB_DCH_CH27/1 -> PDO Transmit DCH_CH27/1
  PWMOUT_CH27/2 -> DTCB_DCL_CH27/1
  DTCB_DCL_CH27/1 -> PDO Transmit DCL_CH27/1
  PWMOUT_CH27/3 -> DTCB_PFH_CH27/1
  DTCB_PFH_CH27/1 -> PDO Transmit PFH_CH27/1
  PWMOUT_CH27/4 -> DTCB_PFL_CH27/1
  DTCB_PFL_CH27/1 -> PDO Transmit PFL_CH27/1
  PWMOUT_DutyCycle_CH28/1 -> PWMOUT_CH28/1
  PWMOUT_Period_CH28/1 -> PWMOUT_CH28/2
  PWMOUT_CH28/1 -> DTCB_DCH_CH28/1
  DTCB_DCH_CH28/1 -> PDO Transmit DCH_CH28/1
  PWMOUT_CH28/2 -> DTCB_DCL_CH28/1
  DTCB_DCL_CH28/1 -> PDO Transmit DCL_CH28/1
  PWMOUT_CH28/3 -> DTCB_PFH_CH28/1
  DTCB_PFH_CH28/1 -> PDO Transmit PFH_CH28/1
  PWMOUT_CH28/4 -> DTCB_PFL_CH28/1
  DTCB_PFL_CH28/1 -> PDO Transmit PFL_CH28/1
  PWMOUT_DutyCycle_CH29/1 -> PWMOUT_CH29/1
  PWMOUT_Period_CH29/1 -> PWMOUT_CH29/2
  PWMOUT_CH29/1 -> DTCB_DCH_CH29/1
  DTCB_DCH_CH29/1 -> PDO Transmit DCH_CH29/1
  PWMOUT_CH29/2 -> DTCB_DCL_CH29/1
  DTCB_DCL_CH29/1 -> PDO Transmit DCL_CH29/1
  PWMOUT_CH29/3 -> DTCB_PFH_CH29/1
  DTCB_PFH_CH29/1 -> PDO Transmit PFH_CH29/1
  PWMOUT_CH29/4 -> DTCB_PFL_CH29/1
  DTCB_PFL_CH29/1 -> PDO Transmit PFL_CH29/1
  PWMOUT_DutyCycle_CH30/1 -> PWMOUT_CH30/1
  PWMOUT_Period_CH30/1 -> PWMOUT_CH30/2
  PWMOUT_CH30/1 -> DTCB_DCH_CH30/1
  DTCB_DCH_CH30/1 -> PDO Transmit DCH_CH30/1
  PWMOUT_CH30/2 -> DTCB_DCL_CH30/1
  DTCB_DCL_CH30/1 -> PDO Transmit DCL_CH30/1
  PWMOUT_CH30/3 -> DTCB_PFH_CH30/1
  DTCB_PFH_CH30/1 -> PDO Transmit PFH_CH30/1
  PWMOUT_CH30/4 -> DTCB_PFL_CH30/1
  DTCB_PFL_CH30/1 -> PDO Transmit PFL_CH30/1
  PWMOUT_DutyCycle_CH31/1 -> PWMOUT_CH31/1
  PWMOUT_Period_CH31/1 -> PWMOUT_CH31/2
  PWMOUT_CH31/1 -> DTCB_DCH_CH31/1
  DTCB_DCH_CH31/1 -> PDO Transmit DCH_CH31/1
  PWMOUT_CH31/2 -> DTCB_DCL_CH31/1
  DTCB_DCL_CH31/1 -> PDO Transmit DCL_CH31/1
  PWMOUT_CH31/3 -> DTCB_PFH_CH31/1
  DTCB_PFH_CH31/1 -> PDO Transmit PFH_CH31/1
  PWMOUT_CH31/4 -> DTCB_PFL_CH31/1
  DTCB_PFL_CH31/1 -> PDO Transmit PFL_CH31/1
  PWMOUT_DutyCycle_CH32/1 -> PWMOUT_CH32/1
  PWMOUT_Period_CH32/1 -> PWMOUT_CH32/2
  PWMOUT_CH32/1 -> DTCB_DCH_CH32/1
  DTCB_DCH_CH32/1 -> PDO Transmit DCH_CH32/1
  PWMOUT_CH32/2 -> DTCB_DCL_CH32/1
  DTCB_DCL_CH32/1 -> PDO Transmit DCL_CH32/1
  PWMOUT_CH32/3 -> DTCB_PFH_CH32/1
  DTCB_PFH_CH32/1 -> PDO Transmit PFH_CH32/1
  PWMOUT_CH32/4 -> DTCB_PFL_CH32/1
  DTCB_PFL_CH32/1 -> PDO Transmit PFL_CH32/1
